simulink model "machine"  (R2023a)
settings: Solver=VariableStepAuto  StartTime=0.0  StopTime=10.0  RelTol=1e-3
values from neighbouring files (symbols this model uses):
  alpha_cu = 3.9 *10^-3    (= 0.0039)    [BLDC_Motor_params_03.m]    (also in DC_Motor_params_01.m; DC_Motor_params_02.m; DC_Motor_params_04.m; DC_Motor_params_05.m)
  b_m1 = .01    (= 0.01)    [DC_Motor_params_01.m]
  b_m2 = .01    (= 0.01)    [DC_Motor_params_02.m]
  b_m3 = .001    (= 0.001)    [BLDC_Motor_params_03.m]
  b_m4 = .3    (= 0.3)    [DC_Motor_params_04.m]
  C_t1 = 19.57    [DC_Motor_params_01.m]
  C_t2 = 66.49    [DC_Motor_params_02.m]
  C_t3 = 50    [BLDC_Motor_params_03.m]
  C_t4 = tao_ts_amb_4/res_term_4    (= 92.0668058455)    [DC_Motor_params_04.m]
  J_eq1 = J_1 + 1/8 * m_1 * d_1^2 / r_1^2    [DC_Motor_params_01.m]
  J_eq2 = J_2 + 1/8 * m_2 * d_2^2 / r_2^2    [DC_Motor_params_02.m]
  J_eq3 = J_3 + 1/8 * m_3 * d_3^2 / r_3^2    [BLDC_Motor_params_03.m]
  J_eq4 = enc_J_4 + J_r4 + J_4 + 1/8 * m_4 * d_4^2 / r_4^2    [DC_Motor_params_04.m]
  K_d1 = 0.022261    [PID_tuning.m]
  K_d2 = 0.07064    [PID_tuning.m]
  K_d3 = 0    [PID_tuning.m]
  K_d4 = 0    [PID_tuning.m]
  k_e1 = 0.25    [DC_Motor_params_01.m]
  k_e2 = 0.56    [DC_Motor_params_02.m]
  k_e3 = 0.3    [BLDC_Motor_params_03.m]
  k_e4 = 0.0156    [DC_Motor_params_04.m]
  K_i1 = 0    [PID_tuning.m]
  K_i2 = 0    [PID_tuning.m]
  K_i3 = 0.4131    [PID_tuning.m]
  K_i4 = 0    [PID_tuning.m]
  K_p1 = 6.6674    [PID_tuning.m]
  K_p2 = 15.5368    [PID_tuning.m]
  K_p3 = 0    [PID_tuning.m]
  K_p4 = 2.44    [PID_tuning.m]
  k_t1 = 0.25    [DC_Motor_params_01.m]
  k_t2 = 0.56    [DC_Motor_params_02.m]
  k_t3 = 0.3    [BLDC_Motor_params_03.m]
  k_t4 = 0.0156    [DC_Motor_params_04.m]
  L_a1 = 7.5*10^-3    (= 0.0075)    [DC_Motor_params_01.m]
  L_a2 = 3*10^-3    (= 0.003)    [DC_Motor_params_02.m]
  L_a3 = 5*10^-3    (= 0.005)    [BLDC_Motor_params_03.m]
  L_a4 = 0.0336*10^-3    (= 3.36e-05)    [DC_Motor_params_04.m]
  r_1 = 25    [DC_Motor_params_01.m]
  r_2 = 5    [DC_Motor_params_02.m]
  r_3 = 2    [BLDC_Motor_params_03.m]
  r_4 = 51    [DC_Motor_params_04.m]
  r_a1_20 = 0.5    [DC_Motor_params_01.m]
  r_a2_20 = 0.25    [DC_Motor_params_02.m]
  r_a3_20 = 0.35    [BLDC_Motor_params_03.m]
  r_a4_20 = 0.108    [DC_Motor_params_04.m]
  res_term_1 = 9.58    [DC_Motor_params_01.m]
  res_term_2 = 3.15    [DC_Motor_params_02.m]
  res_term_3 = 0.1    [BLDC_Motor_params_03.m]
  res_term_4 = 9.58    [DC_Motor_params_04.m]
  T_s0_1 = 20    [use_machine_1.m]    (also in use_solo_motor_1.m)
  T_s0_2 = 20    [use_machine_1.m]    (also in use_solo_motor_2.m)
  T_s4_0 = ans.simulationOut.data(end,3)    [use_solo_motor_4.m]
  theta_m0_1 = 0    [use_machine_1.m]    (also in use_solo_motor_1.m)
  theta_m0_2 = 0    [use_machine_1.m]    (also in use_solo_motor_2.m = 3.14159265359)
  theta_m4_0 = ans.simulationOut.data(end,1)    [use_solo_motor_4.m]
  w_m3_0 = ans.simulationOut.Data(end,1)    [use_solo_motor_3.m]
settings Model: Creator=Usuario  LastModifiedBy=Usuario

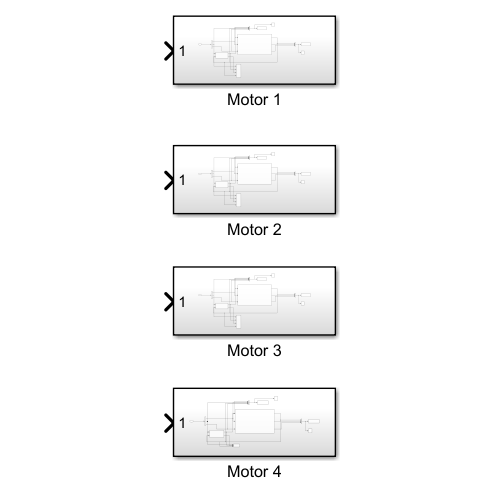
[thumbnail: Simulink's stored preview of the top-level diagram]
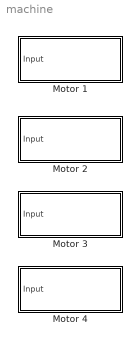
== system machine ==
  Motor 1 : Subsystem
  Motor 2 : Subsystem
  Motor 3 : Subsystem
  Motor 4 : Subsystem

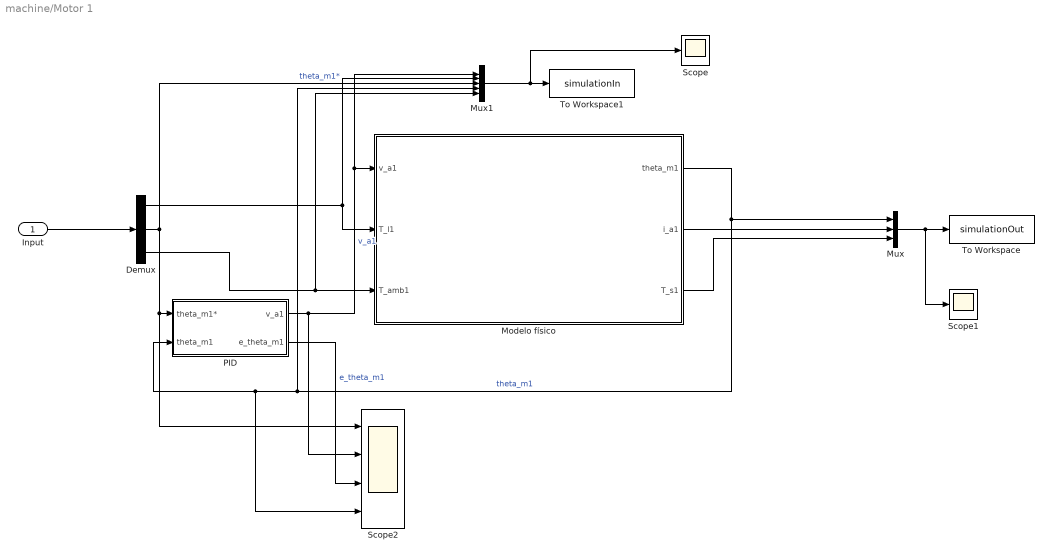
== system machine/Motor 1 ==
  Input : Inport
  Demux : Demux  Outputs=3
  Modelo físico : Subsystem
  Mux : Mux  Inputs=3
  Mux1 : Mux  Inputs=5
  PID : Subsystem
  Scope : Scope
  Scope1 : Scope
  Scope2 : Scope  NumInputPorts=4
  To Workspace : ToWorkspace  VariableName=simulationOut  SaveFormat=Timeseries  SampleTime=-1
  To Workspace1 : ToWorkspace  VariableName=simulationIn  SaveFormat=Timeseries  SampleTime=-1
  wires:
  Modelo físico/1(theta_m1) -> Mux1/4, Scope2/4, PID/2(theta_m1), Mux/1  "theta_m1"
  PID/1(v_a1) -> Scope2/2, Modelo físico/1(v_a1), Mux1/1  "v_a1"
  Demux/1 -> Modelo físico/2(T_l1), Mux1/2
  Mux/1 -> Scope1/1, To Workspace/1
  Mux1/1 -> Scope/1, To Workspace1/1
  Input/1 -> Demux/1
  Modelo físico/2(i_a1) -> Mux/2
  Modelo físico/3(T_s1) -> Mux/3
  Demux/3 -> Mux1/5, Modelo físico/3(T_amb1)
  Demux/2 -> Scope2/1, PID/1(theta_m1*), Mux1/3  "theta_m1*"
  PID/2(e_theta_m1) -> Scope2/3  "e_theta_m1"

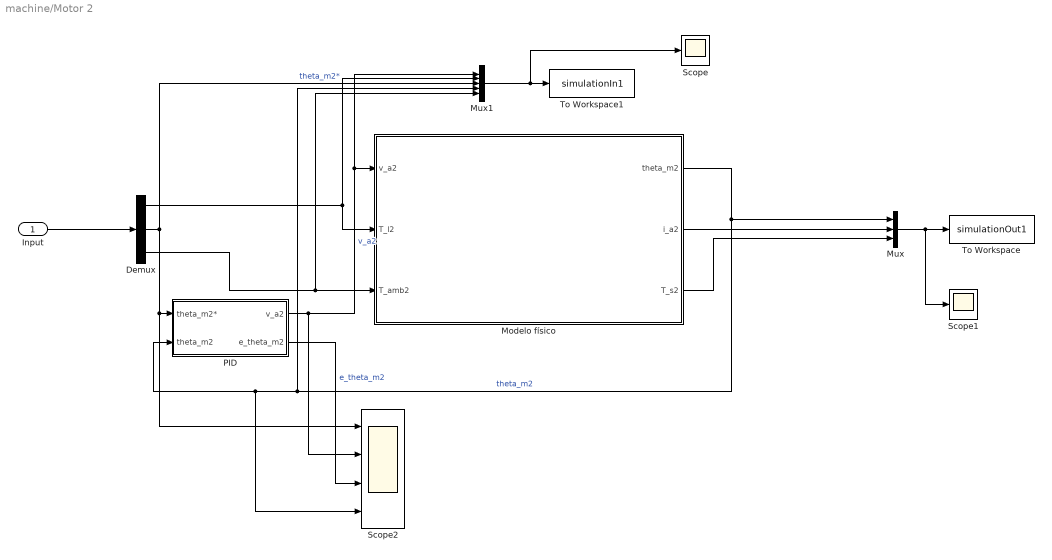
== system machine/Motor 2 ==
  Input : Inport
  Demux : Demux  Outputs=3
  Modelo físico : Subsystem
  Mux : Mux  Inputs=3
  Mux1 : Mux  Inputs=5
  PID : Subsystem
  Scope : Scope
  Scope1 : Scope
  Scope2 : Scope  NumInputPorts=4
  To Workspace : ToWorkspace  VariableName=simulationOut1  SaveFormat=Timeseries  SampleTime=-1
  To Workspace1 : ToWorkspace  VariableName=simulationIn1  SaveFormat=Timeseries  SampleTime=-1
  wires:
  PID/2(e_theta_m2) -> Scope2/3  "e_theta_m2"
  Demux/1 -> Modelo físico/2(T_l2), Mux1/2
  Mux1/1 -> Scope/1, To Workspace1/1
  Demux/3 -> Mux1/5, Modelo físico/3(T_amb2)
  Modelo físico/1(theta_m2) -> Mux1/4, Scope2/4, PID/2(theta_m2), Mux/1  "theta_m2"
  Demux/2 -> Scope2/1, PID/1(theta_m2*), Mux1/3  "theta_m2*"
  Mux/1 -> Scope1/1, To Workspace/1
  Modelo físico/3(T_s2) -> Mux/3
  Modelo físico/2(i_a2) -> Mux/2
  Input/1 -> Demux/1
  PID/1(v_a2) -> Scope2/2, Modelo físico/1(v_a2), Mux1/1  "v_a2"

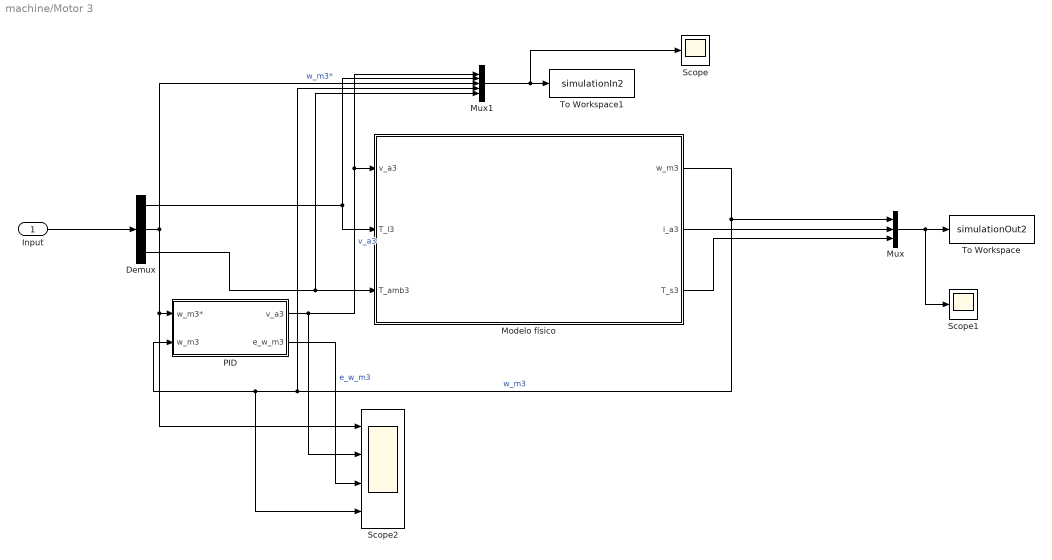
== system machine/Motor 3 ==
  Input : Inport
  Demux : Demux  Outputs=3
  Modelo físico : Subsystem
  Mux : Mux  Inputs=3
  Mux1 : Mux  Inputs=5
  PID : Subsystem
  Scope : Scope
  Scope1 : Scope
  Scope2 : Scope  NumInputPorts=4
  To Workspace : ToWorkspace  VariableName=simulationOut2  SaveFormat=Timeseries  SampleTime=-1
  To Workspace1 : ToWorkspace  VariableName=simulationIn2  SaveFormat=Timeseries  SampleTime=-1
  wires:
  PID/1(v_a3) -> Scope2/2, Modelo físico/1(v_a3), Mux1/1  "v_a3"
  Mux/1 -> Scope1/1, To Workspace/1
  Mux1/1 -> Scope/1, To Workspace1/1
  Input/1 -> Demux/1
  Modelo físico/1(w_m3) -> Mux1/4, Scope2/4, PID/2(w_m3), Mux/1  "w_m3"
  Modelo físico/2(i_a3) -> Mux/2
  Demux/3 -> Mux1/5, Modelo físico/3(T_amb3)
  Demux/2 -> Scope2/1, PID/1(w_m3*), Mux1/3  "w_m3*"
  PID/2(e_w_m3) -> Scope2/3  "e_w_m3"
  Modelo físico/3(T_s3) -> Mux/3
  Demux/1 -> Modelo físico/2(T_l3), Mux1/2

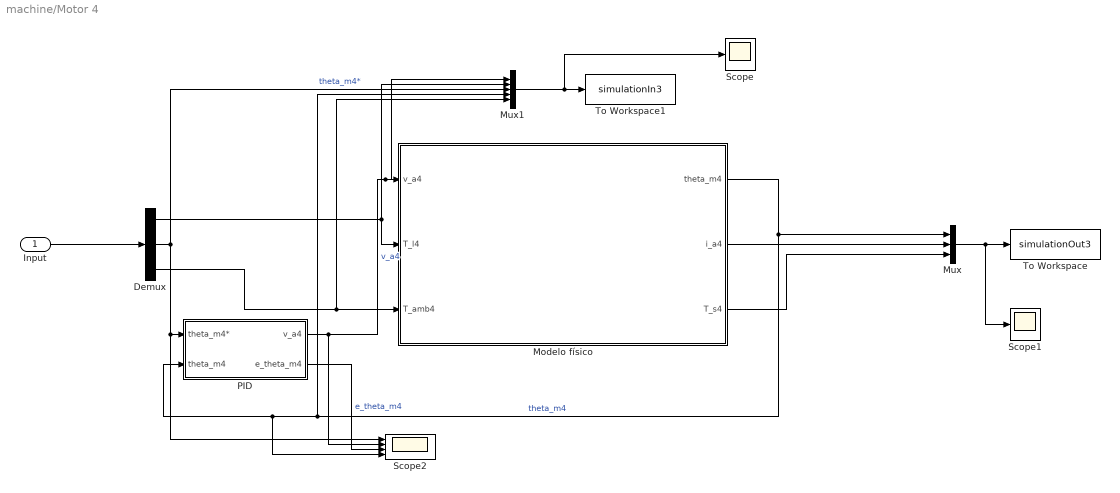
== system machine/Motor 4 ==
  Input : Inport
  Demux : Demux  Outputs=3
  Modelo físico : Subsystem
  Mux : Mux  Inputs=3
  Mux1 : Mux  Inputs=5
  PID : Subsystem
  Scope : Scope
  Scope1 : Scope
  Scope2 : Scope  NumInputPorts=4
  To Workspace : ToWorkspace  VariableName=simulationOut3  SaveFormat=Timeseries  SampleTime=-1
  To Workspace1 : ToWorkspace  VariableName=simulationIn3  SaveFormat=Timeseries  SampleTime=-1
  wires:
  Demux/3 -> Mux1/5, Modelo físico/3(T_amb4)
  Modelo físico/3(T_s4) -> Mux/3
  Mux/1 -> Scope1/1, To Workspace/1
  Demux/1 -> Modelo físico/2(T_l4), Mux1/2
  Modelo físico/2(i_a4) -> Mux/2
  Input/1 -> Demux/1
  Modelo físico/1(theta_m4) -> Mux1/4, Scope2/4, PID/2(theta_m4), Mux/1  "theta_m4"
  Demux/2 -> Scope2/1, PID/1(theta_m4*), Mux1/3  "theta_m4*"
  PID/2(e_theta_m4) -> Scope2/3  "e_theta_m4"
  Mux1/1 -> Scope/1, To Workspace1/1
  PID/1(v_a4) -> Scope2/2, Mux1/1, Modelo físico/1(v_a4)  "v_a4"

== system machine/Motor 1/Modelo físico ==
  v_a1 : Inport
  T_l1 : Inport  Port=2
  T_amb1 : Inport  Port=3
  Subsistema electromagnético : Subsystem
  Subsistema mecánico : Subsystem
  Subsistema térmico : Subsystem
  theta_m1 : Outport
  i_a1 : Outport  Port=2
  T_s1 : Outport  Port=3
  wires:
  Subsistema electromagnético/1(i_a1) -> Subsistema térmico/1(i_a1), Subsistema mecánico/1(i_a1), i_a1/1
  v_a1/1 -> Subsistema electromagnético/1(v_a1)
  T_l1/1 -> Subsistema mecánico/2(T_l1)
  T_amb1/1 -> Subsistema térmico/2(T_amb1)
  Subsistema térmico/1(T_s1) -> T_s1/1
  Subsistema térmico/2(r_a1) -> Subsistema electromagnético/2(r_a1)
  Subsistema mecánico/1(w_m1) -> Subsistema electromagnético/3(w_m1)
  Subsistema mecánico/2(theta_m1) -> theta_m1/1

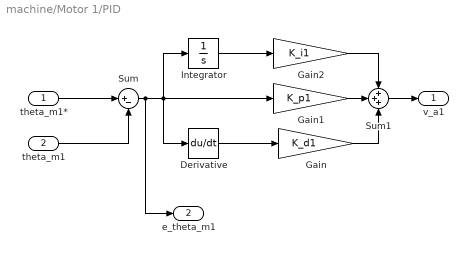
== system machine/Motor 1/PID ==
  theta_m1* : Inport
  theta_m1 : Inport  Port=2
  Derivative : Derivative
  Gain : Gain  Gain=K_d1
  Gain1 : Gain  Gain=K_p1
  Gain2 : Gain  Gain=K_i1
  Integrator : Integrator
  Sum : Sum  Inputs=|+-
  Sum1 : Sum  Inputs=+++
  v_a1 : Outport
  e_theta_m1 : Outport  Port=2
  wires:
  theta_m1*/1 -> Sum/1
  theta_m1/1 -> Sum/2
  Sum/1 -> e_theta_m1/1, Integrator/1, Gain1/1, Derivative/1
  Integrator/1 -> Gain2/1
  Derivative/1 -> Gain/1
  Gain1/1 -> Sum1/2
  Gain2/1 -> Sum1/1
  Sum1/1 -> v_a1/1
  Gain/1 -> Sum1/3

== system machine/Motor 2/Modelo físico ==
  v_a2 : Inport
  T_l2 : Inport  Port=2
  T_amb2 : Inport  Port=3
  Subsistema electromagnético : Subsystem
  Subsistema mecánico : Subsystem
  Subsistema térmico : Subsystem
  theta_m2 : Outport
  i_a2 : Outport  Port=2
  T_s2 : Outport  Port=3
  wires:
  Subsistema electromagnético/1(i_a2) -> Subsistema térmico/1(i_a2), Subsistema mecánico/1(i_a2), i_a2/1
  v_a2/1 -> Subsistema electromagnético/1(v_a2)
  T_l2/1 -> Subsistema mecánico/2(T_l2)
  T_amb2/1 -> Subsistema térmico/2(T_amb2)
  Subsistema térmico/1(T_s2) -> T_s2/1
  Subsistema térmico/2(r_a2) -> Subsistema electromagnético/2(r_a2)
  Subsistema mecánico/1(w_m2) -> Subsistema electromagnético/3(w_m2)
  Subsistema mecánico/2(theta_m2) -> theta_m2/1

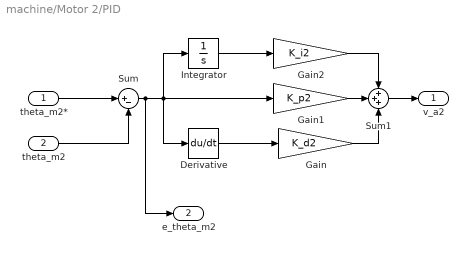
== system machine/Motor 2/PID ==
  theta_m2* : Inport
  theta_m2 : Inport  Port=2
  Derivative : Derivative
  Gain : Gain  Gain=K_d2
  Gain1 : Gain  Gain=K_p2
  Gain2 : Gain  Gain=K_i2
  Integrator : Integrator
  Sum : Sum  Inputs=|+-
  Sum1 : Sum  Inputs=+++
  v_a2 : Outport
  e_theta_m2 : Outport  Port=2
  wires:
  theta_m2*/1 -> Sum/1
  theta_m2/1 -> Sum/2
  Sum/1 -> e_theta_m2/1, Integrator/1, Gain1/1, Derivative/1
  Integrator/1 -> Gain2/1
  Derivative/1 -> Gain/1
  Gain1/1 -> Sum1/2
  Gain2/1 -> Sum1/1
  Sum1/1 -> v_a2/1
  Gain/1 -> Sum1/3

== system machine/Motor 3/Modelo físico ==
  v_a3 : Inport
  T_l3 : Inport  Port=2
  T_amb3 : Inport  Port=3
  Subsistema electromagnético : Subsystem
  Subsistema mecánico : Subsystem
  Subsistema térmico : Subsystem
  w_m3 : Outport
  i_a3 : Outport  Port=2
  T_s3 : Outport  Port=3
  wires:
  Subsistema electromagnético/1(i_a3) -> Subsistema térmico/1(i_a3), Subsistema mecánico/1(i_a3), i_a3/1
  v_a3/1 -> Subsistema electromagnético/1(v_a3)
  T_l3/1 -> Subsistema mecánico/2(T_l3)
  Subsistema mecánico/1(w_m3) -> w_m3/1, Subsistema electromagnético/3(w_m3)
  T_amb3/1 -> Subsistema térmico/2(T_amb3)
  Subsistema térmico/1(T_s3) -> T_s3/1
  Subsistema térmico/2(r_a3) -> Subsistema electromagnético/2(r_a3)

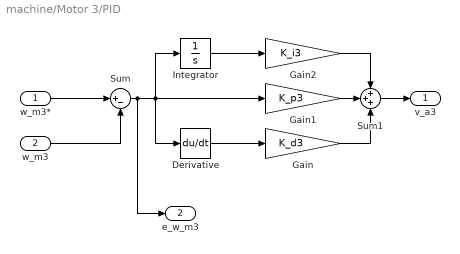
== system machine/Motor 3/PID ==
  w_m3* : Inport
  w_m3 : Inport  Port=2
  Derivative : Derivative
  Gain : Gain  Gain=K_d3
  Gain1 : Gain  Gain=K_p3
  Gain2 : Gain  Gain=K_i3
  Integrator : Integrator
  Sum : Sum  Inputs=|+-
  Sum1 : Sum  Inputs=+++
  v_a3 : Outport
  e_w_m3 : Outport  Port=2
  wires:
  w_m3*/1 -> Sum/1
  w_m3/1 -> Sum/2
  Sum/1 -> e_w_m3/1, Integrator/1, Gain1/1, Derivative/1
  Integrator/1 -> Gain2/1
  Derivative/1 -> Gain/1
  Gain1/1 -> Sum1/2
  Gain2/1 -> Sum1/1
  Sum1/1 -> v_a3/1
  Gain/1 -> Sum1/3

== system machine/Motor 4/Modelo físico ==
  v_a4 : Inport
  T_l4 : Inport  Port=2
  T_amb4 : Inport  Port=3
  Subsistema electromagnético : Subsystem
  Subsistema mecánico : Subsystem
  Subsistema térmico : Subsystem
  theta_m4 : Outport
  i_a4 : Outport  Port=2
  T_s4 : Outport  Port=3
  wires:
  Subsistema mecánico/2(theta_m4) -> theta_m4/1
  Subsistema electromagnético/1(i_a4) -> Subsistema térmico/1(i_a4), Subsistema mecánico/1(i_a4), i_a4/1
  v_a4/1 -> Subsistema electromagnético/1(v_a4)
  T_l4/1 -> Subsistema mecánico/2(T_l4)
  Subsistema mecánico/1(w_m4) -> Subsistema electromagnético/3(w_m4)
  T_amb4/1 -> Subsistema térmico/2(T_amb4)
  Subsistema térmico/1(T_s4) -> T_s4/1
  Subsistema térmico/2(r_a4) -> Subsistema electromagnético/2(r_a4)

== system machine/Motor 4/PID ==
  theta_m4* : Inport
  theta_m4 : Inport  Port=2
  Derivative : Derivative
  Gain : Gain  Gain=K_d4
  Gain1 : Gain  Gain=K_p4
  Gain2 : Gain  Gain=K_i4
  Integrator : Integrator
  Sum : Sum  Inputs=|+-
  Sum1 : Sum  Inputs=+++
  v_a4 : Outport
  e_theta_m4 : Outport  Port=2
  wires:
  theta_m4*/1 -> Sum/1
  theta_m4/1 -> Sum/2
  Sum/1 -> e_theta_m4/1, Integrator/1, Gain1/1, Derivative/1
  Integrator/1 -> Gain2/1
  Derivative/1 -> Gain/1
  Gain1/1 -> Sum1/2
  Gain2/1 -> Sum1/1
  Sum1/1 -> v_a4/1
  Gain/1 -> Sum1/3

== system machine/Motor 1/Modelo físico/Subsistema electromagnético ==
  v_a1 : Inport
  r_a1 : Inport  Port=2
  w_m1 : Inport  Port=3
  Gain1 : Gain  Gain=k_e1
  Gain2 : Gain  Gain=1/L_a1
  Integrator : Integrator
  Product : Product
  Scope : Scope
  Sum : Sum  Inputs=-+-
  i_a1 : Outport
  wires:
  v_a1/1 -> Sum/2
  Integrator/1 -> Product/2, Scope/1, i_a1/1
  Product/1 -> Sum/1
  w_m1/1 -> Gain1/1
  Gain1/1 -> Sum/3
  Sum/1 -> Gain2/1
  Gain2/1 -> Integrator/1
  r_a1/1 -> Product/1

== system machine/Motor 1/Modelo físico/Subsistema mecánico ==
  i_a1 : Inport
  T_l1 : Inport  Port=2
  Gain : Gain  Gain=r_1^2*k_t1
  Gain1 : Gain  Gain=b_m1
  Gain3 : Gain  Gain=1/J_eq1
  Integrator : Integrator
  Integrator1 : Integrator  InitialCondition=theta_m0_1
  Sum : Sum  Inputs=-+-
  w_m1 : Outport
  theta_m1 : Outport  Port=2
  wires:
  i_a1/1 -> Gain/1
  Gain/1 -> Sum/2
  Integrator/1 -> w_m1/1, Gain1/1, Integrator1/1
  Gain1/1 -> Sum/1
  T_l1/1 -> Sum/3
  Gain3/1 -> Integrator/1
  Sum/1 -> Gain3/1
  Integrator1/1 -> theta_m1/1

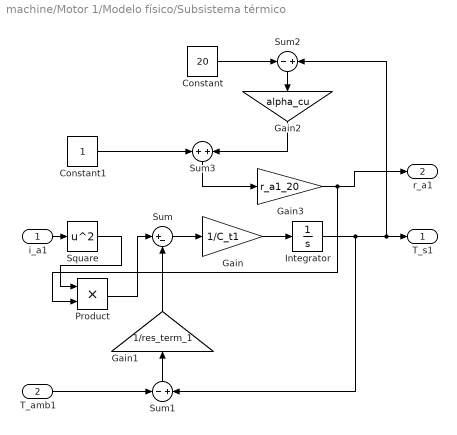
== system machine/Motor 1/Modelo físico/Subsistema térmico ==
  i_a1 : Inport
  T_amb1 : Inport  Port=2
  Constant : Constant  Value=20
  Constant1 : Constant
  Gain : Gain  Gain=1/C_t1
  Gain1 : Gain  Gain=1/res_term_1
  Gain2 : Gain  Gain=alpha_cu
  Gain3 : Gain  Gain=r_a1_20
  Integrator : Integrator  InitialCondition=T_s0_1
  Product : Product
  Square : Math  Operator=square
  Sum : Sum  Inputs=|+-
  Sum1 : Sum  Inputs=-|+
  Sum2 : Sum  Inputs=-|+
  Sum3 : Sum  Inputs=+|+
  T_s1 : Outport
  r_a1 : Outport  Port=2
  wires:
  i_a1/1 -> Square/1
  Sum3/1 -> Gain3/1
  Gain2/1 -> Sum3/2
  Square/1 -> Product/1
  Gain3/1 -> Product/2, r_a1/1
  Sum2/1 -> Gain2/1
  T_amb1/1 -> Sum1/1
  Constant1/1 -> Sum3/1
  Gain/1 -> Integrator/1
  Sum/1 -> Gain/1
  Integrator/1 -> Sum1/2, Sum2/2, T_s1/1
  Constant/1 -> Sum2/1
  Sum1/1 -> Gain1/1
  Gain1/1 -> Sum/2
  Product/1 -> Sum/1

== system machine/Motor 2/Modelo físico/Subsistema electromagnético ==
  v_a2 : Inport
  r_a2 : Inport  Port=2
  w_m2 : Inport  Port=3
  Gain1 : Gain  Gain=k_e2
  Gain2 : Gain  Gain=1/L_a2
  Integrator : Integrator
  Product : Product
  Scope : Scope
  Sum : Sum  Inputs=-+-
  i_a2 : Outport
  wires:
  v_a2/1 -> Sum/2
  Integrator/1 -> Product/2, Scope/1, i_a2/1
  Product/1 -> Sum/1
  w_m2/1 -> Gain1/1
  Gain1/1 -> Sum/3
  Sum/1 -> Gain2/1
  Gain2/1 -> Integrator/1
  r_a2/1 -> Product/1

== system machine/Motor 2/Modelo físico/Subsistema mecánico ==
  i_a2 : Inport
  T_l2 : Inport  Port=2
  Gain : Gain  Gain=r_2^2*k_t2
  Gain1 : Gain  Gain=b_m2
  Gain3 : Gain  Gain=1/J_eq2
  Integrator : Integrator
  Integrator1 : Integrator  InitialCondition=theta_m0_2
  Sum : Sum  Inputs=-+-
  w_m2 : Outport
  theta_m2 : Outport  Port=2
  wires:
  i_a2/1 -> Gain/1
  Gain/1 -> Sum/2
  Integrator/1 -> w_m2/1, Gain1/1, Integrator1/1
  Gain1/1 -> Sum/1
  T_l2/1 -> Sum/3
  Gain3/1 -> Integrator/1
  Sum/1 -> Gain3/1
  Integrator1/1 -> theta_m2/1

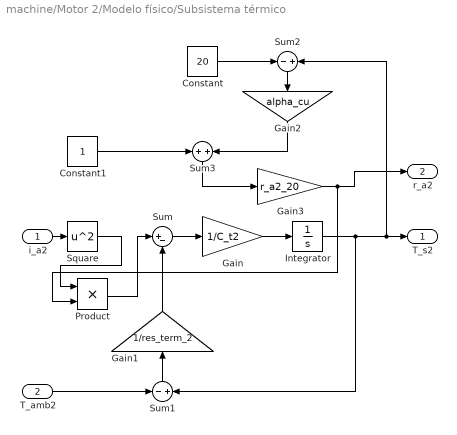
== system machine/Motor 2/Modelo físico/Subsistema térmico ==
  i_a2 : Inport
  T_amb2 : Inport  Port=2
  Constant : Constant  Value=20
  Constant1 : Constant
  Gain : Gain  Gain=1/C_t2
  Gain1 : Gain  Gain=1/res_term_2
  Gain2 : Gain  Gain=alpha_cu
  Gain3 : Gain  Gain=r_a2_20
  Integrator : Integrator  InitialCondition=T_s0_2
  Product : Product
  Square : Math  Operator=square
  Sum : Sum  Inputs=|+-
  Sum1 : Sum  Inputs=-|+
  Sum2 : Sum  Inputs=-|+
  Sum3 : Sum  Inputs=+|+
  T_s2 : Outport
  r_a2 : Outport  Port=2
  wires:
  i_a2/1 -> Square/1
  Sum3/1 -> Gain3/1
  Gain2/1 -> Sum3/2
  Square/1 -> Product/1
  Gain3/1 -> Product/2, r_a2/1
  Sum2/1 -> Gain2/1
  T_amb2/1 -> Sum1/1
  Constant1/1 -> Sum3/1
  Gain/1 -> Integrator/1
  Sum/1 -> Gain/1
  Integrator/1 -> Sum1/2, Sum2/2, T_s2/1
  Constant/1 -> Sum2/1
  Sum1/1 -> Gain1/1
  Gain1/1 -> Sum/2
  Product/1 -> Sum/1

== system machine/Motor 3/Modelo físico/Subsistema electromagnético ==
  v_a3 : Inport
  r_a3 : Inport  Port=2
  w_m3 : Inport  Port=3
  Gain1 : Gain  Gain=k_e3
  Gain2 : Gain  Gain=1/L_a3
  Integrator : Integrator
  Product : Product
  Scope : Scope
  Sum : Sum  Inputs=-+-
  i_a3 : Outport
  wires:
  v_a3/1 -> Sum/2
  Integrator/1 -> Product/2, Scope/1, i_a3/1
  Product/1 -> Sum/1
  w_m3/1 -> Gain1/1
  Gain1/1 -> Sum/3
  Sum/1 -> Gain2/1
  Gain2/1 -> Integrator/1
  r_a3/1 -> Product/1

== system machine/Motor 3/Modelo físico/Subsistema mecánico ==
  i_a3 : Inport
  T_l3 : Inport  Port=2
  Gain : Gain  Gain=r_3^2*k_t3
  Gain1 : Gain  Gain=b_m3
  Gain3 : Gain  Gain=1/J_eq3
  Integrator : Integrator  InitialCondition=w_m3_0
  Integrator1 : Integrator
  Sum : Sum  Inputs=-+-
  w_m3 : Outport
  theta_m3 : Outport  Port=2
  wires:
  i_a3/1 -> Gain/1
  Gain/1 -> Sum/2
  Integrator/1 -> w_m3/1, Gain1/1, Integrator1/1
  Gain1/1 -> Sum/1
  T_l3/1 -> Sum/3
  Gain3/1 -> Integrator/1
  Sum/1 -> Gain3/1
  Integrator1/1 -> theta_m3/1

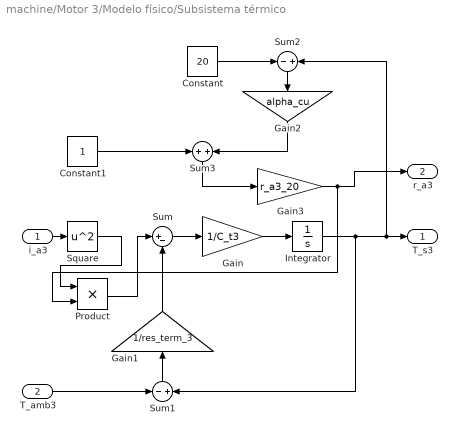
== system machine/Motor 3/Modelo físico/Subsistema térmico ==
  i_a3 : Inport
  T_amb3 : Inport  Port=2
  Constant : Constant  Value=20
  Constant1 : Constant
  Gain : Gain  Gain=1/C_t3
  Gain1 : Gain  Gain=1/res_term_3
  Gain2 : Gain  Gain=alpha_cu
  Gain3 : Gain  Gain=r_a3_20
  Integrator : Integrator
  Product : Product
  Square : Math  Operator=square
  Sum : Sum  Inputs=|+-
  Sum1 : Sum  Inputs=-|+
  Sum2 : Sum  Inputs=-|+
  Sum3 : Sum  Inputs=+|+
  T_s3 : Outport
  r_a3 : Outport  Port=2
  wires:
  i_a3/1 -> Square/1
  Sum3/1 -> Gain3/1
  Gain2/1 -> Sum3/2
  Square/1 -> Product/1
  Gain3/1 -> Product/2, r_a3/1
  Sum2/1 -> Gain2/1
  T_amb3/1 -> Sum1/1
  Constant1/1 -> Sum3/1
  Gain/1 -> Integrator/1
  Sum/1 -> Gain/1
  Integrator/1 -> Sum1/2, Sum2/2, T_s3/1
  Constant/1 -> Sum2/1
  Sum1/1 -> Gain1/1
  Gain1/1 -> Sum/2
  Product/1 -> Sum/1

== system machine/Motor 4/Modelo físico/Subsistema electromagnético ==
  v_a4 : Inport
  r_a4 : Inport  Port=2
  w_m4 : Inport  Port=3
  Gain1 : Gain  Gain=k_e4
  Gain2 : Gain  Gain=1/L_a4
  Integrator : Integrator
  Product : Product
  Scope : Scope
  Sum : Sum  Inputs=-+-
  i_a4 : Outport
  wires:
  v_a4/1 -> Sum/2
  Integrator/1 -> Product/2, Scope/1, i_a4/1
  Product/1 -> Sum/1
  w_m4/1 -> Gain1/1
  Gain1/1 -> Sum/3
  Sum/1 -> Gain2/1
  Gain2/1 -> Integrator/1
  r_a4/1 -> Product/1

== system machine/Motor 4/Modelo físico/Subsistema mecánico ==
  i_a4 : Inport
  T_l4 : Inport  Port=2
  Gain : Gain  Gain=r_4^2*k_t4
  Gain1 : Gain  Gain=b_m4
  Gain3 : Gain  Gain=1/J_eq4
  Integrator : Integrator
  Integrator1 : Integrator  InitialCondition=theta_m4_0
  Sum : Sum  Inputs=-+-
  w_m4 : Outport
  theta_m4 : Outport  Port=2
  wires:
  i_a4/1 -> Gain/1
  Gain/1 -> Sum/2
  Integrator/1 -> w_m4/1, Gain1/1, Integrator1/1
  Gain1/1 -> Sum/1
  T_l4/1 -> Sum/3
  Gain3/1 -> Integrator/1
  Sum/1 -> Gain3/1
  Integrator1/1 -> theta_m4/1

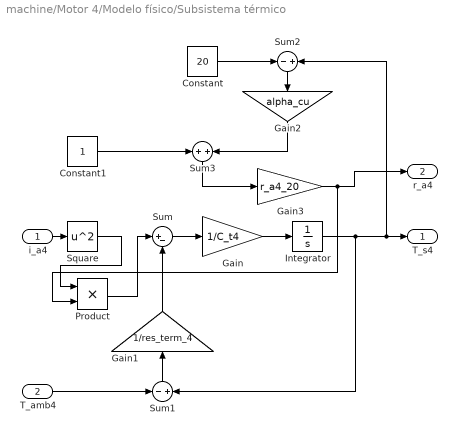
== system machine/Motor 4/Modelo físico/Subsistema térmico ==
  i_a4 : Inport
  T_amb4 : Inport  Port=2
  Constant : Constant  Value=20
  Constant1 : Constant
  Gain : Gain  Gain=1/C_t4
  Gain1 : Gain  Gain=1/res_term_4
  Gain2 : Gain  Gain=alpha_cu
  Gain3 : Gain  Gain=r_a4_20
  Integrator : Integrator  InitialCondition=T_s4_0
  Product : Product
  Square : Math  Operator=square
  Sum : Sum  Inputs=|+-
  Sum1 : Sum  Inputs=-|+
  Sum2 : Sum  Inputs=-|+
  Sum3 : Sum  Inputs=+|+
  T_s4 : Outport
  r_a4 : Outport  Port=2
  wires:
  i_a4/1 -> Square/1
  Sum3/1 -> Gain3/1
  Gain2/1 -> Sum3/2
  Square/1 -> Product/1
  Gain3/1 -> Product/2, r_a4/1
  Sum2/1 -> Gain2/1
  T_amb4/1 -> Sum1/1
  Constant1/1 -> Sum3/1
  Gain/1 -> Integrator/1
  Sum/1 -> Gain/1
  Integrator/1 -> Sum1/2, Sum2/2, T_s4/1
  Constant/1 -> Sum2/1
  Sum1/1 -> Gain1/1
  Gain1/1 -> Sum/2
  Product/1 -> Sum/1
